simulink model "Tphase"  (R2017a)
settings: Solver=FixedStepDiscrete  StartTime=0.0  StopTime=0.125 - 5e-5  MaxStep=1e-4  RelTol=1e-3
undefined symbols (not defined in the file): D1, Delta
libraries: powerlib x57, auto_lib x2
settings Model: Creator=ioanna  LastModifiedBy=ioanna

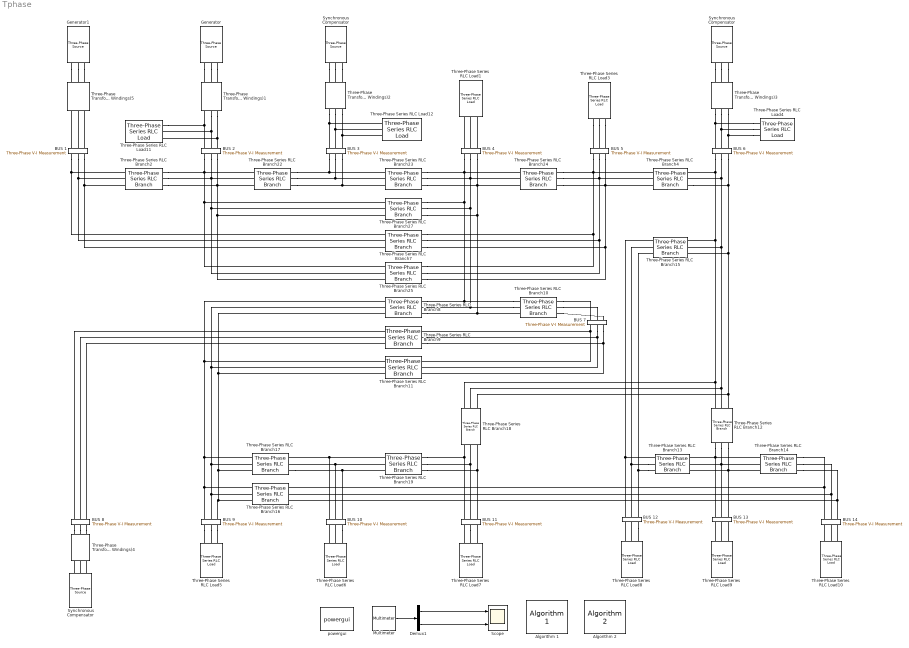
== system Tphase ==
  " Generator" : powerlib/Electrical Sources/Three-Phase Source  InternalConnection=Yg  VoltagePhases=off  Voltage=1.045  PhaseAngle=-30  Voltage_phases=[25e3 25e3 25e3]/sqrt(3)  PhaseAngles_phases=[0 -120 +120]  Frequency=50  NonIdealSource=on  SpecifyImpedance=on  Resistance=0.8929  Inductance=16.58e-3  ShortCircuitLevel=10  BaseVoltage=1  XRratio=1  BusType=PV  Pref=0.4  Qref=0  Prefabc=[10e3, 10e3, 10e3]  Qrefabc=[0, 0, 0]  Qmin=-0.4  Qmax=0.5
  " Generator1" : powerlib/Electrical Sources/Three-Phase Source  InternalConnection=Yg  VoltagePhases=off  Voltage=1.06  PhaseAngle=-30  Voltage_phases=[25e3 25e3 25e3]/sqrt(3)  PhaseAngles_phases=[0 -120 +120]  Frequency=50  NonIdealSource=on  SpecifyImpedance=on  Resistance=0.8929  Inductance=16.58e-3  ShortCircuitLevel=10  BaseVoltage=1  XRratio=1  BusType=PQ  Pref=2.324  Qref=-0.169  Prefabc=[10e3, 10e3, 10e3]  Qrefabc=[0, 0, 0]  Qmin=0  Qmax=0
  Algorithm 1 : auto_lib/Algorithm 1  SystemSampleTime=-1
      settings: SourceProductName=Auto_Design_Framework
  Algorithm 2 : auto_lib/Algorithm 2  SystemSampleTime=-1
      settings: SourceProductName=Auto_Design_Framework
  BUS {1..14} (14 alike) : powerlib/Measurements/Three-Phase V-I Measurement  VoltageMeasurement=no  SetLabelV=off  LabelV=Vabc  Vpu=off  VpuLL=off  CurrentMeasurement=no  SetLabelI=off  LabelI=Iabc  Ipu=off  Pbase=100e6  Vbase=500e3  OutputType=Complex  PhasorSimulation=off  PSBequivalent=0
  Demux1 : Demux  Outputs=2
  Multimeter : powerlib/Measurements/Multimeter  PhasorSimulation=off  OutputType=Complex  sel=[1 2 3 4 5 6]  L=6  Gain=[1 1 1 1 1 1]  yselected={'Uag: Three-Phase Series RLC Load10','Ubg: Three-Phase Series RLC Load10','Ucg: Three-Phase Series RLC Load10','Iag: Three-Phase Series RLC Load10','Ibg: Three-Phase Series RLC Load10','Icg: Three-Phase Series RLC Load10'};  PSBOutputType=1  PSBequivalent=0  AxesSetting=[0,0.1,-100,100]  Display=0  SavedBlockNames=-11
  Scope : Scope  NumInputPorts=2
  Synchronous Compensator : powerlib/Electrical Sources/Three-Phase Source  InternalConnection=Yg  VoltagePhases=off  Voltage=1.09  PhaseAngle=-30  Voltage_phases=[25e3 25e3 25e3]/sqrt(3)  PhaseAngles_phases=[0 -120 +120]  Frequency=50  NonIdealSource=on  SpecifyImpedance=on  Resistance=0.8929  Inductance=16.58e-3  ShortCircuitLevel=10  BaseVoltage=1  XRratio=1  BusType=PV  Pref=0  Qref=0  Prefabc=[10e3, 10e3, 10e3]  Qrefabc=[0, 0, 0]  Qmin=-0.06  Qmax=0.24
  Synchronous Compensator : powerlib/Electrical Sources/Three-Phase Source  InternalConnection=Yg  VoltagePhases=off  Voltage=1.01  PhaseAngle=-30  Voltage_phases=[25e3 25e3 25e3]/sqrt(3)  PhaseAngles_phases=[0 -120 +120]  Frequency=50  NonIdealSource=on  SpecifyImpedance=on  Resistance=0.8929  Inductance=16.58e-3  ShortCircuitLevel=10  BaseVoltage=1  XRratio=1  BusType=PV  Pref=0  Qref=23.4e6  Prefabc=[10e3, 10e3, 10e3]  Qrefabc=[0, 0, 0]  Qmin=0  Qmax=0.4
  "Synchronous Compensator " : powerlib/Electrical Sources/Three-Phase Source  InternalConnection=Yg  VoltagePhases=off  Voltage=1.07  PhaseAngle=-30  Voltage_phases=[25e3 25e3 25e3]/sqrt(3)  PhaseAngles_phases=[0 -120 +120]  Frequency=50  NonIdealSource=on  SpecifyImpedance=on  Resistance=0.8929  Inductance=16.58e-3  ShortCircuitLevel=10  BaseVoltage=1  XRratio=1  BusType=PV  Pref=0  Qref=23.4e6  Prefabc=[10e3, 10e3, 10e3]  Qrefabc=[0, 0, 0]  Qmin=-0.06  Qmax=0.24
  Three-Phase Series RLC Branch10 : powerlib/Elements/Three-Phase Series RLC Branch  LConnTagsString=A|B|C  RConnTagsString=A|B|C  BranchType=L  Resistance=1  Inductance=0.20912/(2*pi*50)  Capacitance=1e-6  Measurements=None
  Three-Phase Series RLC Branch11 : powerlib/Elements/Three-Phase Series RLC Branch  LConnTagsString=A|B|C  RConnTagsString=A|B|C  BranchType=L  Resistance=1  Inductance=0.11001/(2*pi*50)  Capacitance=1e-6  Measurements=None
  Three-Phase Series RLC Branch12 : powerlib/Elements/Three-Phase Series RLC Branch  LConnTagsString=A|B|C  RConnTagsString=A|B|C  BranchType=RL  Resistance=0.06615  Inductance=0.13027/(2*pi*50)  Capacitance=1e-6  Measurements=None
  Three-Phase Series RLC Branch13 : powerlib/Elements/Three-Phase Series RLC Branch  LConnTagsString=A|B|C  RConnTagsString=A|B|C  BranchType=RL  Resistance=0.22092  Inductance=0.19988/(2*pi*50)  Capacitance=1e-6  Measurements=None
  Three-Phase Series RLC Branch14 : powerlib/Elements/Three-Phase Series RLC Branch  LConnTagsString=A|B|C  RConnTagsString=A|B|C  BranchType=RL  Resistance=0.17093  Inductance=0.34802/(2*pi*50)  Capacitance=1e-6  Measurements=None
  Three-Phase Series RLC Branch15 : powerlib/Elements/Three-Phase Series RLC Branch  LConnTagsString=A|B|C  RConnTagsString=A|B|C  BranchType=RL  Resistance=0.12291  Inductance=0.25581/(2*pi*50)  Capacitance=1e-6  Measurements=None
  Three-Phase Series RLC Branch16 : powerlib/Elements/Three-Phase Series RLC Branch  LConnTagsString=A|B|C  RConnTagsString=A|B|C  BranchType=RL  Resistance=0.12711  Inductance=0.27038/(2*pi*50)  Capacitance=1e-6  Measurements=None
  Three-Phase Series RLC Branch17 : powerlib/Elements/Three-Phase Series RLC Branch  LConnTagsString=A|B|C  RConnTagsString=A|B|C  BranchType=RL  Resistance=0.03181  Inductance=0.08450/(2*pi*50)  Capacitance=1e-6  Measurements=None
  Three-Phase Series RLC Branch18 : powerlib/Elements/Three-Phase Series RLC Branch  LConnTagsString=A|B|C  RConnTagsString=A|B|C  BranchType=RL  Resistance=0.09498  Inductance=0.1989/(2*pi*50)  Capacitance=1e-6  Measurements=None
  Three-Phase Series RLC Branch19 : powerlib/Elements/Three-Phase Series RLC Branch  LConnTagsString=A|B|C  RConnTagsString=A|B|C  BranchType=RL  Resistance=0.08205  Inductance=0.19207/(2*pi*50)  Capacitance=1e-6  Measurements=None
  Three-Phase Series RLC Branch2 : powerlib/Elements/Three-Phase Series RLC Branch  LConnTagsString=A|B|C  RConnTagsString=A|B|C  BranchType=RLC  Resistance=0.01938  Inductance=0.05917/(2*pi*50)  Capacitance=0.01/0.0528/(2*pi*50)  Measurements=None
  Three-Phase Series RLC Branch22 : powerlib/Elements/Three-Phase Series RLC Branch  LConnTagsString=A|B|C  RConnTagsString=A|B|C  BranchType=RLC  Resistance=0.04699  Inductance=0.19797/(2*pi*50)  Capacitance=0.01/0.0438/(2*pi*50)  Measurements=None
  Three-Phase Series RLC Branch23 : powerlib/Elements/Three-Phase Series RLC Branch  LConnTagsString=A|B|C  RConnTagsString=A|B|C  BranchType=RLC  Resistance=0.06701  Inductance=0.17103/(2*pi*50)  Capacitance=0.01/0.0346/(2*pi*50)  Measurements=None
  Three-Phase Series RLC Branch24 : powerlib/Elements/Three-Phase Series RLC Branch  LConnTagsString=A|B|C  RConnTagsString=A|B|C  BranchType=RLC  Resistance=0.01335  Inductance=0.04211/(2*pi*50)  Capacitance=0.01/0.0128/(2*pi*50)  Measurements=None
  Three-Phase Series RLC Branch25 : powerlib/Elements/Three-Phase Series RLC Branch  LConnTagsString=A|B|C  RConnTagsString=A|B|C  BranchType=RLC  Resistance=0.05695  Inductance=0.17388/(2*pi*50)  Capacitance=0.01/0.0340/(2*pi*50)  Measurements=None
  Three-Phase Series RLC Branch27 : powerlib/Elements/Three-Phase Series RLC Branch  LConnTagsString=A|B|C  RConnTagsString=A|B|C  BranchType=RLC  Resistance=0.05811  Inductance=0.17632/(2*pi*50)  Capacitance=0.01/0.0374/(2*pi*50)  Measurements=None
  Three-Phase Series RLC Branch4 : powerlib/Elements/Three-Phase Series RLC Branch  LConnTagsString=A|B|C  RConnTagsString=A|B|C  BranchType=L  Resistance=1  Inductance=0.25202/(2*pi*50)  Capacitance=1e-6  Measurements=None
  Three-Phase Series RLC Branch7 : powerlib/Elements/Three-Phase Series RLC Branch  LConnTagsString=A|B|C  RConnTagsString=A|B|C  BranchType=RLC  Resistance=0.05403  Inductance=0.22304/(2*pi*50)  Capacitance=0.01/0.0492/(2*pi*50)  Measurements=None
  Three-Phase Series RLC Branch8 : powerlib/Elements/Three-Phase Series RLC Branch  LConnTagsString=A|B|C  RConnTagsString=A|B|C  BranchType=L  Resistance=1  Inductance=0.55618/(2*pi*50)  Capacitance=1e-6  Measurements=None
  Three-Phase Series RLC Branch9 : powerlib/Elements/Three-Phase Series RLC Branch  LConnTagsString=A|B|C  RConnTagsString=A|B|C  BranchType=L  Resistance=1  Inductance=0.17615/(2*pi*50)  Capacitance=1e-6  Measurements=None
  Three-Phase Series RLC Load1 : powerlib/Elements/Three-Phase Series RLC Load  LConnTagsString=A|B|C  Configuration=Y (grounded)  NominalVoltage=1  Vabc=[1e3 1e3 1e3]  Vabcp=[1e3 1e3 1e3]  NominalFrequency=50  UnbalancedPower=off  ActivePower=0.478  InductivePower=0  CapacitivePower=0.039  Pabc=[10e3 9e3 11e3]  QLabc=[100 90 110]  QCabc=[100 90 110]  Pabcp=[10e3 9e3 11e3]  QLabcp=[100 90 110]  QCabcp=[100 90 110]  Measurements=None  LoadType=constant PQ
  Three-Phase Series RLC Load10 : powerlib/Elements/Three-Phase Series RLC Load  LConnTagsString=A|B|C  Configuration=Y (grounded)  NominalVoltage=1  Vabc=[1e3 1e3 1e3]  Vabcp=[1e3 1e3 1e3]  NominalFrequency=50  UnbalancedPower=off  ActivePower=0.149  InductivePower=0.050  CapacitivePower=0  Pabc=[10e3 9e3 11e3]  QLabc=[100 90 110]  QCabc=[100 90 110]  Pabcp=[10e3 9e3 11e3]  QLabcp=[100 90 110]  QCabcp=[100 90 110]  Measurements=Branch voltages and currents  LoadType=constant Z
  Three-Phase Series RLC Load11 : powerlib/Elements/Three-Phase Series RLC Load  LConnTagsString=A|B|C  Configuration=Y (grounded)  NominalVoltage=1  Vabc=[1e3 1e3 1e3]  Vabcp=[1e3 1e3 1e3]  NominalFrequency=50  UnbalancedPower=off  ActivePower=0.217  InductivePower=0.127  CapacitivePower=0  Pabc=[10e3 9e3 11e3]  QLabc=[100 90 110]  QCabc=[100 90 110]  Pabcp=[10e3 9e3 11e3]  QLabcp=[100 90 110]  QCabcp=[100 90 110]  Measurements=None  LoadType=constant PQ
  Three-Phase Series RLC Load12 : powerlib/Elements/Three-Phase Series RLC Load  LConnTagsString=A|B|C  Configuration=Y (grounded)  NominalVoltage=1  Vabc=[1e3 1e3 1e3]  Vabcp=[1e3 1e3 1e3]  NominalFrequency=50  UnbalancedPower=off  ActivePower=0.942  InductivePower=0.191  CapacitivePower=0  Pabc=[10e3 9e3 11e3]  QLabc=[100 90 110]  QCabc=[100 90 110]  Pabcp=[10e3 9e3 11e3]  QLabcp=[100 90 110]  QCabcp=[100 90 110]  Measurements=None  LoadType=constant PQ
  Three-Phase Series RLC Load3 : powerlib/Elements/Three-Phase Series RLC Load  LConnTagsString=A|B|C  Configuration=Y (grounded)  NominalVoltage=1  Vabc=[1e3 1e3 1e3]  Vabcp=[1e3 1e3 1e3]  NominalFrequency=50  UnbalancedPower=off  ActivePower=0.076  InductivePower=0.016  CapacitivePower=0  Pabc=[10e3 9e3 11e3]  QLabc=[100 90 110]  QCabc=[100 90 110]  Pabcp=[10e3 9e3 11e3]  QLabcp=[100 90 110]  QCabcp=[100 90 110]  Measurements=None  LoadType=constant PQ
  Three-Phase Series RLC Load4 : powerlib/Elements/Three-Phase Series RLC Load  LConnTagsString=A|B|C  Configuration=Y (grounded)  NominalVoltage=1  Vabc=[1e3 1e3 1e3]  Vabcp=[1e3 1e3 1e3]  NominalFrequency=50  UnbalancedPower=off  ActivePower=0.112  InductivePower=0.075  CapacitivePower=0  Pabc=[10e3 9e3 11e3]  QLabc=[100 90 110]  QCabc=[100 90 110]  Pabcp=[10e3 9e3 11e3]  QLabcp=[100 90 110]  QCabcp=[100 90 110]  Measurements=None  LoadType=constant PQ
  Three-Phase Series RLC Load5 : powerlib/Elements/Three-Phase Series RLC Load  LConnTagsString=A|B|C  Configuration=Y (grounded)  NominalVoltage=1  Vabc=[1e3 1e3 1e3]  Vabcp=[1e3 1e3 1e3]  NominalFrequency=50  UnbalancedPower=off  ActivePower=0.295  InductivePower=0.166  CapacitivePower=0  Pabc=[10e3 9e3 11e3]  QLabc=[100 90 110]  QCabc=[100 90 110]  Pabcp=[10e3 9e3 11e3]  QLabcp=[100 90 110]  QCabcp=[100 90 110]  Measurements=None  LoadType=constant PQ
  Three-Phase Series RLC Load6 : powerlib/Elements/Three-Phase Series RLC Load  LConnTagsString=A|B|C  Configuration=Y (grounded)  NominalVoltage=1  Vabc=[1e3 1e3 1e3]  Vabcp=[1e3 1e3 1e3]  NominalFrequency=50  UnbalancedPower=off  ActivePower=0.09  InductivePower=0.058  CapacitivePower=0  Pabc=[10e3 9e3 11e3]  QLabc=[100 90 110]  QCabc=[100 90 110]  Pabcp=[10e3 9e3 11e3]  QLabcp=[100 90 110]  QCabcp=[100 90 110]  Measurements=None  LoadType=constant PQ
  Three-Phase Series RLC Load7 : powerlib/Elements/Three-Phase Series RLC Load  LConnTagsString=A|B|C  Configuration=Y (grounded)  NominalVoltage=1  Vabc=[1e3 1e3 1e3]  Vabcp=[1e3 1e3 1e3]  NominalFrequency=50  UnbalancedPower=off  ActivePower=0.035  InductivePower=0.018  CapacitivePower=0  Pabc=[10e3 9e3 11e3]  QLabc=[100 90 110]  QCabc=[100 90 110]  Pabcp=[10e3 9e3 11e3]  QLabcp=[100 90 110]  QCabcp=[100 90 110]  Measurements=None  LoadType=constant PQ
  Three-Phase Series RLC Load8 : powerlib/Elements/Three-Phase Series RLC Load  LConnTagsString=A|B|C  Configuration=Y (grounded)  NominalVoltage=1  Vabc=[1e3 1e3 1e3]  Vabcp=[1e3 1e3 1e3]  NominalFrequency=50  UnbalancedPower=off  ActivePower=0.061  InductivePower=0.016  CapacitivePower=0  Pabc=[10e3 9e3 11e3]  QLabc=[100 90 110]  QCabc=[100 90 110]  Pabcp=[10e3 9e3 11e3]  QLabcp=[100 90 110]  QCabcp=[100 90 110]  Measurements=None  LoadType=constant PQ
  Three-Phase Series RLC Load9 : powerlib/Elements/Three-Phase Series RLC Load  LConnTagsString=A|B|C  Configuration=Y (grounded)  NominalVoltage=1  Vabc=[1e3 1e3 1e3]  Vabcp=[1e3 1e3 1e3]  NominalFrequency=50  UnbalancedPower=off  ActivePower=0.135  InductivePower=0.058  CapacitivePower=0  Pabc=[10e3 9e3 11e3]  QLabc=[100 90 110]  QCabc=[100 90 110]  Pabcp=[10e3 9e3 11e3]  QLabcp=[100 90 110]  QCabcp=[100 90 110]  Measurements=None  LoadType=constant PQ
  Three-Phase Transformer (Two Windings)1 : powerlib/Elements/Three-Phase Transformer (Two Windings)  Winding1Connection=Delta (D1)  Winding2Connection=Yg  CoreType=Three single-phase transformers  SetSaturation=off  Hysteresis=off  DataFile='hysteresis'  SetInitialFlux=off  Measurements=None  UNITS=pu  NominalPower=[ 1 , 50 ]  Winding1=[ 1.045 , 0.002 , 0.08 ]  Winding2=[ 1.045 , 0.002 , 0.08 ]  Rm=500  Lm=500  L0=0.5  Saturation=[ 0,0 ; 0.0024,1.2 ; 1.0,1.52 ]  InitialFluxes=[ 0.8 , -0.8 , 0.7 ]  MoreParameters=off  BreakLoop=off  DataType=off  TransfoNumber=1
  Three-Phase Transformer (Two Windings)2 : powerlib/Elements/Three-Phase Transformer (Two Windings)  Winding1Connection=Delta (D1)  Winding2Connection=Yg  CoreType=Three single-phase transformers  SetSaturation=off  Hysteresis=off  DataFile='hysteresis'  SetInitialFlux=off  Measurements=None  UNITS=pu  NominalPower=[ 1 , 50 ]  Winding1=[ 1.01 , 0.002 , 0.08 ]  Winding2=[ 1.01 , 0.002 , 0.08 ]  Rm=500  Lm=500  L0=0.5  Saturation=[ 0,0 ; 0.0024,1.2 ; 1.0,1.52 ]  InitialFluxes=[ 0.8 , -0.8 , 0.7 ]  MoreParameters=off  BreakLoop=off  DataType=off  TransfoNumber=1
  Three-Phase Transformer (Two Windings)3 : powerlib/Elements/Three-Phase Transformer (Two Windings)  Winding1Connection=Delta (D1)  Winding2Connection=Yg  CoreType=Three single-phase transformers  SetSaturation=off  Hysteresis=off  DataFile='hysteresis'  SetInitialFlux=off  Measurements=None  UNITS=pu  NominalPower=[ 1 , 50 ]  Winding1=[ 1.07 , 0.002 , 0.08 ]  Winding2=[ 1.07 , 0.002 , 0.08 ]  Rm=500  Lm=500  L0=0.5  Saturation=[ 0,0 ; 0.0024,1.2 ; 1.0,1.52 ]  InitialFluxes=[ 0.8 , -0.8 , 0.7 ]  MoreParameters=off  BreakLoop=off  DataType=off  TransfoNumber=1
  Three-Phase Transformer (Two Windings)4 : powerlib/Elements/Three-Phase Transformer (Two Windings)  Winding1Connection=Yg  Winding2Connection=Delta (D1)  CoreType=Three single-phase transformers  SetSaturation=off  Hysteresis=off  DataFile='hysteresis'  SetInitialFlux=off  Measurements=None  UNITS=pu  NominalPower=[ 1 , 50 ]  Winding1=[ 1.09 , 0.002 , 0.08]  Winding2=[1.09 , 0.002 , 0.08]  Rm=500  Lm=500  L0=0.5  Saturation=[0 0;0.0023999 1.2;1 1.52]  InitialFluxes=[0.80002 -0.80002 0.69999]  MoreParameters=off  BreakLoop=off  DataType=off  TransfoNumber=1
  Three-Phase Transformer (Two Windings)5 : powerlib/Elements/Three-Phase Transformer (Two Windings)  Winding1Connection=Delta (D1)  Winding2Connection=Yg  CoreType=Three single-phase transformers  SetSaturation=off  Hysteresis=off  DataFile='hysteresis'  SetInitialFlux=off  Measurements=None  UNITS=pu  NominalPower=[ 1, 50 ]  Winding1=[ 1.06 , 0.002 , 0.08 ]  Winding2=[ 1.06 , 0.002 , 0.08 ]  Rm=500  Lm=500  L0=0.5  Saturation=[ 0,0 ; 0.0024,1.2 ; 1.0,1.52 ]  InitialFluxes=[ 0.8 , -0.8 , 0.7 ]  MoreParameters=off  BreakLoop=off  DataType=off  TransfoNumber=1
  powergui : powerlib/powergui  Priority=1  SimulationMode=Discrete  SampleTime=50e-6  frequency=60  Iterations=50  frequencyindice=50  Pbase=100e6  ErrMax=1e-4  UnitsV=kV  UnitsW=MW  buscounter=0  FunctionMessages=off  echomessages=off  EnableUseOfTLC=off  CurrentSourceSwitches=off  DisableSnubberDevices=off  DisableRonSwitches=off  DisableVfSwitches=off  DisplayEquations=off  SolverType=Tustin  Interpol=off  ExternalGateDelay=off  methode=off  Ts=100  x0status=zero  SPID=on  SwTol=0  HookPort=off  RestoreLinks=warning  ResistiveCurrentMeasurement=off  Frange=[0:2:500]  Ylog=off  Xlog=on  ShowGrid=off  save=off  variable=ZData  structure=logsout  ZoomFFT=off  StartTime=0.0  cycles=1  DisplayStyle=1  fundamental=60  FreqAxis=off  MaxFrequency=1000  frequencyindicesteady=1  RmsSteady=1  display=off
  wires:
  Multimeter/1 -> Demux1/1
  Demux1/1 -> Scope/1
  Demux1/2 -> Scope/2
  connections:
  Three-Phase Series RLC Branch14/LConn1 -- Three-Phase Series RLC Branch16/LConn1 -- BUS 14/LConn1
  Three-Phase Series RLC Load4/LConn2 -- BUS 6/LConn2 -- Three-Phase Transformer (Two Windings)3/RConn2
  Three-Phase Series RLC Branch12/LConn1 -- Three-Phase Series RLC Branch18/LConn1 -- Three-Phase Series RLC Branch15/LConn1 -- Three-Phase Series RLC Branch4/RConn1 -- BUS 6/RConn1
  Three-Phase Series RLC Branch25/RConn1 -- Three-Phase Series RLC Branch7/RConn1 -- Three-Phase Series RLC Branch24/RConn1 -- Three-Phase Series RLC Branch4/LConn1 -- BUS 5/RConn1
  Three-Phase Series RLC Load4/LConn3 -- Three-Phase Transformer (Two Windings)3/RConn3 -- BUS 6/LConn3
  Three-Phase Series RLC Branch16/RConn3 -- BUS 9/LConn3 -- Three-Phase Series RLC Branch8/LConn3 -- Three-Phase Series RLC Branch11/RConn3 -- Three-Phase Series RLC Branch17/RConn3
  Three-Phase Transformer (Two Windings)2/RConn2 -- Three-Phase Series RLC Load12/LConn2 -- BUS 3/LConn2
  Three-Phase Series RLC Branch23/LConn1 -- Three-Phase Series RLC Branch22/RConn1 -- BUS 3/RConn1
  Three-Phase Series RLC Branch2/RConn3 -- Three-Phase Series RLC Branch22/LConn3 -- Three-Phase Series RLC Branch27/LConn3 -- Three-Phase Series RLC Branch25/LConn3 -- BUS 2/RConn3
  Three-Phase Series RLC Branch11/LConn2 -- Three-Phase Series RLC Branch9/RConn2 -- BUS 7/RConn2
  Three-Phase Series RLC Branch12/RConn2 -- Three-Phase Series RLC Branch14/RConn2 -- BUS 13/LConn2 -- Three-Phase Series RLC Branch13/LConn2
  BUS 1/RConn3 -- Three-Phase Series RLC Branch2/LConn3 -- Three-Phase Series RLC Branch7/LConn3
  Three-Phase Series RLC Branch9/RConn1 -- BUS 7/RConn1 -- Three-Phase Series RLC Branch11/LConn1
  Three-Phase Series RLC Branch27/LConn1 -- Three-Phase Series RLC Branch25/LConn1 -- Three-Phase Series RLC Branch2/RConn1 -- Three-Phase Series RLC Branch22/LConn1 -- BUS 2/RConn1
  Three-Phase Series RLC Branch14/LConn2 -- Three-Phase Series RLC Branch16/LConn2 -- BUS 14/LConn2
  Three-Phase Series RLC Branch25/RConn2 -- Three-Phase Series RLC Branch7/RConn2 -- Three-Phase Series RLC Branch24/RConn2 -- Three-Phase Series RLC Branch4/LConn2 -- BUS 5/RConn2
  Three-Phase Series RLC Branch24/LConn3 -- Three-Phase Series RLC Branch23/RConn3 -- Three-Phase Series RLC Branch27/RConn3 -- Three-Phase Series RLC Branch8/RConn3 -- Three-Phase Series RLC Branch10/LConn3 -- BUS 4/RConn3
  BUS 11/LConn3 -- Three-Phase Series RLC Branch18/RConn3 -- Three-Phase Series RLC Branch19/RConn3
  Three-Phase Series RLC Branch25/RConn3 -- Three-Phase Series RLC Branch7/RConn3 -- Three-Phase Series RLC Branch24/RConn3 -- Three-Phase Series RLC Branch4/LConn3 -- BUS 5/RConn3
  Three-Phase Series RLC Branch19/LConn3 -- Three-Phase Series RLC Branch17/LConn3 -- BUS 10/LConn3
  Three-Phase Series RLC Branch10/LConn2 -- Three-Phase Series RLC Branch8/RConn2 -- Three-Phase Series RLC Branch27/RConn2 -- Three-Phase Series RLC Branch23/RConn2 -- BUS 4/RConn2 -- Three-Phase Series RLC Branch24/LConn2
  Three-Phase Series RLC Branch19/LConn1 -- BUS 10/LConn1 -- Three-Phase Series RLC Branch17/LConn1
  Three-Phase Series RLC Branch11/LConn3 -- Three-Phase Series RLC Branch9/RConn3 -- BUS 7/RConn3
  Three-Phase Series RLC Branch10/LConn1 -- Three-Phase Series RLC Branch8/RConn1 -- Three-Phase Series RLC Branch27/RConn1 -- Three-Phase Series RLC Branch23/RConn1 -- BUS 4/RConn1 -- Three-Phase Series RLC Branch24/LConn1
  Three-Phase Series RLC Branch18/LConn3 -- Three-Phase Series RLC Branch12/LConn3 -- Three-Phase Series RLC Branch15/LConn3 -- Three-Phase Series RLC Branch4/RConn3 -- BUS 6/RConn3
  Three-Phase Transformer (Two Windings)2/RConn1 -- Three-Phase Series RLC Load12/LConn1 -- BUS 3/LConn1
  Three-Phase Series RLC Branch22/LConn2 -- BUS 2/RConn2 -- Three-Phase Series RLC Branch2/RConn2 -- Three-Phase Series RLC Branch27/LConn2 -- Three-Phase Series RLC Branch25/LConn2
  BUS 1/RConn2 -- Three-Phase Series RLC Branch7/LConn2 -- Three-Phase Series RLC Branch2/LConn2
  Three-Phase Transformer (Two Windings)1/RConn2 -- BUS 2/LConn2 -- Three-Phase Series RLC Load11/LConn2
  Three-Phase Series RLC Branch14/RConn1 -- Three-Phase Series RLC Branch12/RConn1 -- BUS 13/LConn1 -- Three-Phase Series RLC Branch13/LConn1
  Three-Phase Transformer (Two Windings)1/RConn3 -- BUS 2/LConn3 -- Three-Phase Series RLC Load11/LConn3
  Three-Phase Series RLC Branch23/LConn2 -- Three-Phase Series RLC Branch22/RConn2 -- BUS 3/RConn2
  Three-Phase Series RLC Branch15/LConn2 -- Three-Phase Series RLC Branch12/LConn2 -- Three-Phase Series RLC Branch18/LConn2 -- Three-Phase Series RLC Branch4/RConn2 -- BUS 6/RConn2
  Three-Phase Series RLC Branch14/RConn3 -- Three-Phase Series RLC Branch12/RConn3 -- BUS 13/LConn3 -- Three-Phase Series RLC Branch13/LConn3
  Three-Phase Series RLC Branch17/RConn1 -- Three-Phase Series RLC Branch8/LConn1 -- Three-Phase Series RLC Branch11/RConn1 -- Three-Phase Series RLC Branch16/RConn1 -- BUS 9/LConn1
  Three-Phase Series RLC Branch8/LConn2 -- Three-Phase Series RLC Branch11/RConn2 -- BUS 9/LConn2 -- Three-Phase Series RLC Branch16/RConn2 -- Three-Phase Series RLC Branch17/RConn2
  Three-Phase Series RLC Branch14/LConn3 -- Three-Phase Series RLC Branch16/LConn3 -- BUS 14/LConn3
  Three-Phase Series RLC Branch13/RConn1 -- Three-Phase Series RLC Branch15/RConn1 -- BUS 12/LConn1
  BUS 1/RConn1 -- Three-Phase Series RLC Branch7/LConn1 -- Three-Phase Series RLC Branch2/LConn1
  Three-Phase Series RLC Branch13/RConn3 -- Three-Phase Series RLC Branch15/RConn3 -- BUS 12/LConn3
  Three-Phase Series RLC Load4/LConn1 -- BUS 6/LConn1 -- Three-Phase Transformer (Two Windings)3/RConn1
  Three-Phase Series RLC Branch23/LConn3 -- Three-Phase Series RLC Branch22/RConn3 -- BUS 3/RConn3
  BUS 11/LConn1 -- Three-Phase Series RLC Branch18/RConn1 -- Three-Phase Series RLC Branch19/RConn1
  BUS 11/LConn2 -- Three-Phase Series RLC Branch18/RConn2 -- Three-Phase Series RLC Branch19/RConn2
  Three-Phase Series RLC Branch13/RConn2 -- Three-Phase Series RLC Branch15/RConn2 -- BUS 12/LConn2
  Three-Phase Transformer (Two Windings)2/RConn3 -- Three-Phase Series RLC Load12/LConn3 -- BUS 3/LConn3
  Three-Phase Series RLC Load11/LConn1 -- Three-Phase Transformer (Two Windings)1/RConn1 -- BUS 2/LConn1
  Three-Phase Series RLC Branch19/LConn2 -- BUS 10/LConn2 -- Three-Phase Series RLC Branch17/LConn2
  Three-Phase Series RLC Load6/LConn1 -- BUS 10/RConn1
  Three-Phase Series RLC Load10/LConn2 -- BUS 14/RConn2
  BUS 9/RConn2 -- Three-Phase Series RLC Load5/LConn2
  Three-Phase Series RLC Load9/LConn2 -- BUS 13/RConn2
  BUS 8/RConn1 -- Three-Phase Transformer (Two Windings)4/LConn1
  Three-Phase Series RLC Branch9/LConn2 -- BUS 8/LConn2
  BUS 12/RConn3 -- Three-Phase Series RLC Load8/LConn3
  Three-Phase Series RLC Load7/LConn3 -- BUS 11/RConn3
  Three-Phase Series RLC Load10/LConn3 -- BUS 14/RConn3
  Three-Phase Series RLC Load8/LConn1 -- BUS 12/RConn1
  Three-Phase Series RLC Load9/LConn1 -- BUS 13/RConn1
  Three-Phase Series RLC Branch10/RConn1 -- BUS 7/LConn1
  Three-Phase Series RLC Load3/LConn2 -- BUS 5/LConn2
  BUS 4/LConn2 -- Three-Phase Series RLC Load1/LConn2
  Synchronous Compensator/RConn1 -- Three-Phase Transformer (Two Windings)4/RConn1
  BUS 4/LConn3 -- Three-Phase Series RLC Load1/LConn3
  Three-Phase Series RLC Load8/LConn2 -- BUS 12/RConn2
  " Generator1"/RConn1 -- Three-Phase Transformer (Two Windings)5/LConn1
  BUS 9/RConn3 -- Three-Phase Series RLC Load5/LConn3
  "Synchronous Compensator "/RConn2 -- Three-Phase Transformer (Two Windings)3/LConn2
  BUS 8/LConn1 -- Three-Phase Series RLC Branch9/LConn1
  Synchronous Compensator/RConn3 -- Three-Phase Transformer (Two Windings)4/RConn3
  BUS 1/LConn3 -- Three-Phase Transformer (Two Windings)5/RConn3
  " Generator1"/RConn3 -- Three-Phase Transformer (Two Windings)5/LConn3
  Three-Phase Series RLC Branch10/RConn3 -- BUS 7/LConn3
  " Generator"/RConn1 -- Three-Phase Transformer (Two Windings)1/LConn1
  BUS 1/LConn2 -- Three-Phase Transformer (Two Windings)5/RConn2
  " Generator"/RConn3 -- Three-Phase Transformer (Two Windings)1/LConn3
  Synchronous Compensator/RConn2 -- Three-Phase Transformer (Two Windings)2/LConn2
  Three-Phase Series RLC Load10/LConn1 -- BUS 14/RConn1
  BUS 8/RConn3 -- Three-Phase Transformer (Two Windings)4/LConn3
  " Generator1"/RConn2 -- Three-Phase Transformer (Two Windings)5/LConn2
  BUS 10/RConn3 -- Three-Phase Series RLC Load6/LConn3
  Three-Phase Series RLC Load9/LConn3 -- BUS 13/RConn3
  " Generator"/RConn2 -- Three-Phase Transformer (Two Windings)1/LConn2
  Synchronous Compensator/RConn3 -- Three-Phase Transformer (Two Windings)2/LConn3
  "Synchronous Compensator "/RConn1 -- Three-Phase Transformer (Two Windings)3/LConn1
  Synchronous Compensator/RConn1 -- Three-Phase Transformer (Two Windings)2/LConn1
  "Synchronous Compensator "/RConn3 -- Three-Phase Transformer (Two Windings)3/LConn3
  Three-Phase Series RLC Load3/LConn3 -- BUS 5/LConn3
  BUS 1/LConn1 -- Three-Phase Transformer (Two Windings)5/RConn1
  Three-Phase Series RLC Load6/LConn2 -- BUS 10/RConn2
  Three-Phase Series RLC Branch10/RConn2 -- BUS 7/LConn2
  BUS 8/LConn3 -- Three-Phase Series RLC Branch9/LConn3
  BUS 4/LConn1 -- Three-Phase Series RLC Load1/LConn1
  BUS 8/RConn2 -- Three-Phase Transformer (Two Windings)4/LConn2
  Three-Phase Series RLC Load3/LConn1 -- BUS 5/LConn1
  BUS 11/RConn2 -- Three-Phase Series RLC Load7/LConn2
  Three-Phase Series RLC Load7/LConn1 -- BUS 11/RConn1
  BUS 9/RConn1 -- Three-Phase Series RLC Load5/LConn1
  Synchronous Compensator/RConn2 -- Three-Phase Transformer (Two Windings)4/RConn2
